simulink library "ad_high_scalar"  (R2017a)
settings: Solver=VariableStepAuto  StartTime=0.0  StopTime=10.0  RelTol=1e-3
libraries: autodiff x9
settings Model: Creator=eruffaldi  LastModifiedBy=eruffaldi

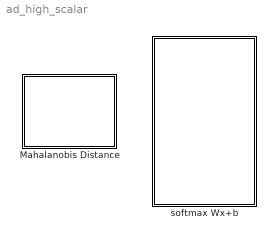
== system ad_high_scalar ==
  " Mahalanobis Distance " : Subsystem
  softmax Wx+b : Subsystem

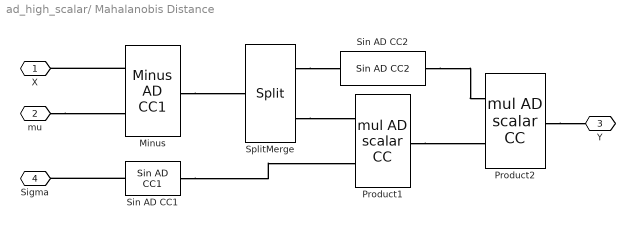
== system ad_high_scalar/ Mahalanobis Distance  ==
  Minus : autodiff/Minus AD CC1
      settings: SourceProductName=AutoDiff
  Product1 : autodiff/mul AD scalar CC
      settings: SourceProductName=AutoDiff
  Product2 : autodiff/mul AD scalar CC
      settings: SourceProductName=AutoDiff
  Sin AD CC1 : autodiff/Sin AD CC1  SystemSampleTime=-1
      settings: SourceProductName=AutoDiff
  Sin AD CC2 : autodiff/Sin AD CC2  SystemSampleTime=-1
      settings: SourceProductName=AutoDiff
  SplitMerge : autodiff/Split  SystemSampleTime=-1
      settings: SourceProductName=AutoDiff
  X : PMIOPort  Port=1  Side=Left
  mu : PMIOPort  Port=2  Side=Left
  Y : PMIOPort  Port=3  Side=Right
  Sigma : PMIOPort  Port=4  Side=Left
  connections:
  Product2/RConn1 -- Y/RConn1
  Minus/LConn1 -- X/RConn1
  mu/RConn1 -- Minus/LConn2
  Sin AD CC1/LConn1 -- Sigma/RConn1
  Sin AD CC1/RConn1 -- Product1/LConn2
  Minus/RConn1 -- SplitMerge/LConn1
  SplitMerge/RConn2 -- Product1/LConn1
  SplitMerge/RConn1 -- Sin AD CC2/LConn1
  Sin AD CC2/RConn1 -- Product2/LConn1
  Product1/RConn1 -- Product2/LConn2

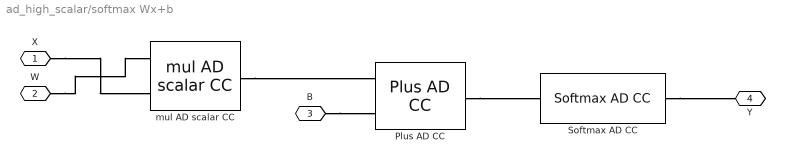
== system ad_high_scalar/softmax Wx+b ==
  Plus AD CC : autodiff/Plus AD CC
      settings: SourceProductName=AutoDiff
  Softmax AD CC : autodiff/Softmax AD CC  SystemSampleTime=-1
      settings: SourceProductName=AutoDiff
  mul AD scalar CC : autodiff/mul AD scalar CC
      settings: SourceProductName=AutoDiff
  X : PMIOPort  Port=1  Side=Left
  W : PMIOPort  Port=2  Side=Left
  B : PMIOPort  Port=3  Side=Left
  Y : PMIOPort  Port=4  Side=Right
  connections:
  Softmax AD CC/RConn1 -- Y/RConn1
  Plus AD CC/RConn1 -- Softmax AD CC/LConn1
  mul AD scalar CC/RConn1 -- Plus AD CC/LConn1
  B/RConn1 -- Plus AD CC/LConn2
  X/RConn1 -- mul AD scalar CC/LConn2
  W/RConn1 -- mul AD scalar CC/LConn1
